simulink model "testRT"  (R2018b)
settings: Solver=FixedStepAuto  StartTime=0.0  StopTime=20  FixedStep=0.0125  RelTol=1e-3  EnableMultiTasking=on
settings Model: Creator=barthal  LastModifiedBy=barthal
settings SolverCC: PositivePriorityOrder=on
settings DataIOCC: Decimation=5  SaveFormat=StructureWithTime
settings OptimizationCC: EnhancedBackFolding=on  PassReuseOutputArgsAs=Individual arguments  MaxStackSize=64  OptimizeBlockOrder=speed  DifferentSizesBufferReuse=on  OptimizationCustomize=off
settings DebuggingCC: ParameterTunabilityLossMsg=error
settings HardwareCC: ProdBitPerPointer=32  ProdBitPerSizeT=32  ProdBitPerPtrDiffT=32  ProdLargestAtomicInteger=Long  ProdLargestAtomicFloat=Double  ProdWordSize=32  ProdHWDeviceType=ARM Compatible->ARM Cortex
settings ModelReferenceCC: ModelReferenceNumInstancesAllowed=Single
settings RTWCC: SystemTargetFile=ert.tlc  HardwareBoard=Raspberry Pi  TLCOptions="-aInlineSetEventsForThisBaseRateFcn=TLC_FALSE -aSuppressMultiTaskScheduler=TLC_FALSE  -aRateBasedStepFcn=0"  GenCodeOnly=on  TemplateMakefile=ert_default_tmf  GenerateReport=on  Toolchain=GNU GCC Raspberry Pi  BuildConfiguration=Faster Runs  IncludeHyperlinkInReport=on  LaunchReport=on  TargetLang=C++  GenerateTraceInfo=on  GenerateTraceReport=on  GenerateTraceReportSl=on  GenerateTraceReportSf=on  GenerateTraceReportEml=on
settings CodeAppCC: ForceParamTrailComments=on  IgnoreCustomStorageClasses=off  OperatorAnnotations=on  SimulinkDataObjDesc=on  SFDataObjDesc=on  InsertBlockDesc=on
settings ERTTargetCC: TargetLangStandard=C++03 (ISO)  MatFileLogging=on  MultiInstanceERTCode=on  CodeInterfacePackaging=C++ class  SupportVariableSizeSignals=on  MultiInstanceErrorCode=Warning  RootIOFormat=Structure reference

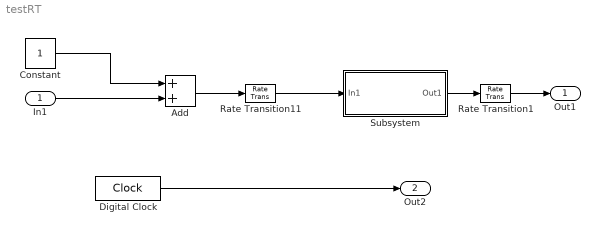
== system testRT ==
  In1 : Inport  OutDataTypeStr=int32  PortDimensions=1
  Add : Sum
  Constant : Constant
  Digital Clock : DigitalClock  SampleTime=0.0125
  Rate Transition1 : RateTransition  OutPortSampleTime=0.0125
  Rate Transition11 : RateTransition  OutPortSampleTime=0.025
  Subsystem : Subsystem  TreatAsAtomicUnit=on  SystemSampleTime=0.025
  Out1 : Outport
  Out2 : Outport  Port=2
  wires:
  In1/1 -> Add/2
  Add/1 -> Rate Transition11/1
  Subsystem/1(Out1) -> Rate Transition1/1
  Constant/1 -> Add/1
  Digital Clock/1 -> Out2/1
  Rate Transition11/1 -> Subsystem/1(In1)
  Rate Transition1/1 -> Out1/1

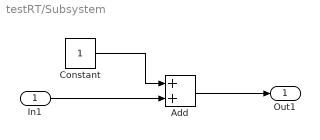
== system testRT/Subsystem ==
  In1 : Inport
  Add : Sum
  Constant : Constant
  Out1 : Outport
  wires:
  Constant/1 -> Add/1
  In1/1 -> Add/2
  Add/1 -> Out1/1
